simulink model "zw"  (Simulink 6.1)
settings: Solver=ode4  SolverMode=SingleTasking  StartTime=0.0  StopTime=15  FixedStep=0.001  RelTol=1e-3
values from neighbouring files (symbols this model uses):
  K_alpha2az = Z_alpha*177    (= 84.96)    [Design_posun.m]    (also in abcdef.m)
  M_alpha = -1.94    [Design_posun.m]    (also in abcdef.m)
  M_dlte = 1.3    [Design_posun.m]    (also in abcdef.m)
  M_q = 0.11    [Design_posun.m]    (also in abcdef.m)
  Z_alpha = 0.48    [Design_posun.m]    (also in abcdef.m)
  Z_dlte = 0    [Design_posun.m]    (also in abcdef.m)
undefined symbols (not defined in the file or in its folder): kaz, kq
settings Model: LastModifiedBy=ybstrong
settings DebuggingCC: SolverPrmCheckMsg=warning

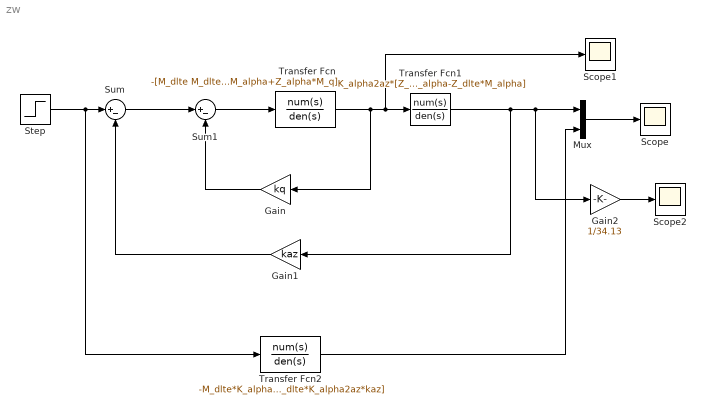
== system zw ==
  Gain : Gain  Orientation=left  Gain=kq
  Gain1 : Gain  Orientation=left  Gain=kaz
  Gain2 : Gain  Gain=1/34.13
  Mux : Mux  Inputs=2
  Scope : Scope
  Scope1 : Scope
  Scope2 : Scope
      settings: SaveName=ScopeData2
  Step : Step  Time=0  SampleTime=0
  Sum : Sum  Inputs=|+-
  Sum1 : Sum  Inputs=|+-
  Transfer Fcn : TransferFcn  Numerator=-[M_dlte M_dlte*Z_alpha-Z_dlte*M_alpha]  Denominator=[1 Z_alpha+M_q M_alpha+Z_alpha*M_q]
  Transfer Fcn1 : TransferFcn  Numerator=K_alpha2az*[Z_dlte M_dlte+Z_dlte*M_q]  Denominator=[M_dlte M_dlte*Z_alpha-Z_dlte*M_alpha]
  Transfer Fcn2 : TransferFcn  Numerator=-M_dlte*K_alpha2az  Denominator=[1 Z_alpha+M_q-M_dlte*kq M_alpha+Z_alpha*M_q-M_dlte*Z_alpha*kq-M_dlte*K_alpha2az*kaz]
  wires:
  Step/1 -> Sum/1, Transfer Fcn2/1
  Sum/1 -> Sum1/1
  Sum1/1 -> Transfer Fcn/1
  Transfer Fcn/1 -> Gain/1, Transfer Fcn1/1, Scope1/1
  Gain/1 -> Sum1/2
  Transfer Fcn1/1 -> Gain1/1, Mux/1, Gain2/1
  Gain1/1 -> Sum/2
  Transfer Fcn2/1 -> Mux/2
  Mux/1 -> Scope/1
  Gain2/1 -> Scope2/1
